simulink model "pd_lq_dob"  (Simulink 4.00)
settings: Solver=ode45  StartTime=0.0  StopTime=100.0  RelTol=1e-3
values from neighbouring files (symbols this model uses):
  B = 2.3006    [para_pdwithfriction.m]    (also in paradob.m)
  F_step = 0.1    [paradob.m]
  J = 2.7721    [para_pdwithfriction.m]    (also in paradob.m)
  Kp = 1    [para_pdwithfriction.m]    (also in paradob.m = 1.5)
  Kv = 0.02    [para_pdwithfriction.m]    (also in paradob.m)
  lqden = [ 1, -1.99971715402018,0.99972174296204,0,0,0]    [para_pdwithfriction.m]    (also in paradob.m = [1,-1.99630389598519,0.99631099777277,0,0,0])
  lqnum = 1000000*[1.50819599815358,-4.52194815122789,3.01001451018836,3.01970189465354,-4.52263469082776,1.50667043906476]    [para_pdwithfriction.m]    (also in paradob.m = 1000000*[0.99631443754708,-2.98490658969623,1.98438945750937)
  ts = 0.001    [para_pdwithfriction.m]    (also in paradob.m)
undefined symbols (not defined in the file or in its folder): g2den, g2num, qzden, qznum
libraries: simulink3 x1
settings Model: LastModifiedBy=liuyuan1  MaxDataPoints=100000  ExtModeTrigMode=oneshot  ExtModeArmWhenConnect=off

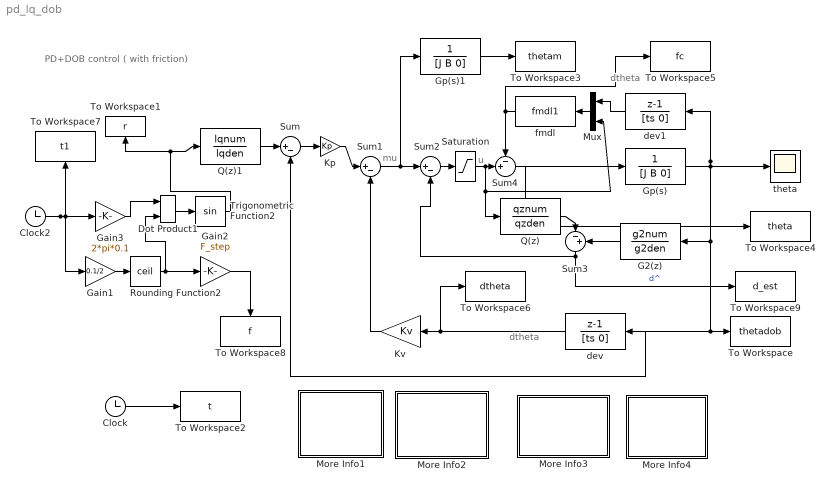
== system pd_lq_dob ==
  note: dtheta
  note: u
  note: PD+DOB control ( with friction)
  note: dtheta
  note: mu
  " Kv" : Gain  Orientation=left  Gain=Kv  Multiplication=Element-wise(K.*u)  SaturateOnIntegerOverflow=on
  Clock : Clock
      settings: DisplayTime=off  Decimation=10
  Clock2 : Clock
      settings: Decimation=10
  Dot Product1 : simulink3/Math/Dot Product
  G2(z) : DiscreteTransferFcn  Orientation=left  Numerator=g2num  Denominator=g2den  SampleTime=0.001  Realization=auto
      settings: RTWStateStorageClass=Auto
  Gain1 : Gain  Gain=0.1/2  Multiplication=Element-wise(K.*u)  SaturateOnIntegerOverflow=on
  Gain2 : Gain  Gain=F_step  Multiplication=Element-wise(K.*u)  SaturateOnIntegerOverflow=on
  Gain3 : Gain  Gain=2*pi*0.1  Multiplication=Element-wise(K.*u)  SaturateOnIntegerOverflow=on
  Gp(s) : TransferFcn  Numerator=[0 0 1]  Denominator=[J B 0]  AbsoluteTolerance=auto  Realization=auto
  Gp(s)1 : TransferFcn  Numerator=[0 0 1]  Denominator=[J B 0]  AbsoluteTolerance=auto  Realization=auto
  "Kp " : Gain  Gain=Kp  Multiplication=Element-wise(K.*u)  SaturateOnIntegerOverflow=on
  More Info1 : Subsystem
      settings: OpenFcn=eval(['paradob']);  RTWFcnNameOpts=Auto  RTWFileNameOpts=Auto
      mask Display: disp('Double click\nhere for\nload parameters')
  More Info2 : Subsystem
      settings: OpenFcn=eval(['postdobwithfriction']);  RTWFcnNameOpts=Auto  RTWFileNameOpts=Auto
      mask Display: disp('Double click\nhere for plot')
  More Info3 : Subsystem
      settings: OpenFcn=eval(['test_freq']);  RTWFcnNameOpts=Auto  RTWFileNameOpts=Auto
      mask Display: disp('Double click\nhere for \ncompute frequency')
  More Info4 : Subsystem
      settings: OpenFcn=eval(['bode_plot']);  RTWFcnNameOpts=Auto  RTWFileNameOpts=Auto
      mask Display: disp('Double click\nhere for \ndraw bode')
  Mux : Mux  Orientation=left  Inputs=2
  Q(z) : DiscreteTransferFcn  Numerator=qznum  Denominator=qzden  SampleTime=0.001  Realization=auto
      settings: RTWStateStorageClass=Auto
  Q(z)1 : DiscreteTransferFcn  Numerator=lqnum  Denominator=lqden  SampleTime=0.001  Realization=auto
      settings: RTWStateStorageClass=Auto
  Rounding Function2 : Rounding  Operator=ceil
  Saturation : Saturate  UpperLimit=10  LowerLimit=-10  LinearizeAsGain=on
  Sum : Sum  Inputs=|+-  SaturateOnIntegerOverflow=on
  Sum1 : Sum  Inputs=|+-  SaturateOnIntegerOverflow=on
  Sum2 : Sum  Inputs=|+-  SaturateOnIntegerOverflow=on
  Sum3 : Sum  Orientation=down  Inputs=|-+  SaturateOnIntegerOverflow=on
  Sum4 : Sum  Inputs=-+|  SaturateOnIntegerOverflow=on
  To Workspace : ToWorkspace  VariableName=thetadob  SampleTime=-1  SaveFormat=Array
      settings: MaxDataPoints=100000
  To Workspace1 : ToWorkspace  VariableName=r  SampleTime=-1  SaveFormat=Array
      settings: Orientation=up  MaxDataPoints=100000
  To Workspace2 : ToWorkspace  VariableName=t  SampleTime=-1  SaveFormat=Array
      settings: MaxDataPoints=100000
  To Workspace3 : ToWorkspace  VariableName=thetam  SampleTime=-1  SaveFormat=Array
      settings: MaxDataPoints=100000
  To Workspace4 : ToWorkspace  VariableName=theta  SampleTime=-1  SaveFormat=Array
      settings: MaxDataPoints=100000
  To Workspace5 : ToWorkspace  VariableName=fc  SampleTime=-1  SaveFormat=Array
      settings: MaxDataPoints=100000
  To Workspace6 : ToWorkspace  VariableName=dtheta  SampleTime=-1  SaveFormat=Array
      settings: MaxDataPoints=100000
  To Workspace7 : ToWorkspace  VariableName=t1  SampleTime=-1  SaveFormat=Array
      settings: Orientation=up
  To Workspace8 : ToWorkspace  VariableName=f  SampleTime=-1  SaveFormat=Array
      settings: Orientation=down  MaxDataPoints=100000
  To Workspace9 : ToWorkspace  VariableName=d_est  SampleTime=-1  SaveFormat=Array
      settings: MaxDataPoints=100000
  Trigonometric Function2 : Trigonometry  Operator=sin  OutputSignalType=auto
  dev : DiscreteTransferFcn  Orientation=left  Numerator=[1 -1]  Denominator=[ts 0]  SampleTime=0.001  Realization=auto
      settings: RTWStateStorageClass=Auto
  dev1 : DiscreteTransferFcn  Orientation=left  Numerator=[1 -1]  Denominator=[ts 0]  SampleTime=0.001  Realization=auto
      settings: RTWStateStorageClass=Auto
  fmdl : MATLABFcn  Orientation=left  MATLABFcn=fmdl1  OutputDimensions=-1  OutputSignalType=auto  Output1D=on
      settings: AttributesFormatString=fmdl2
  theta : Scope
      settings: TimeRange=auto  YMin=-1.5  YMax=1.5  SaveToWorkspace=off  SaveName=ScopeData  LimitDataPoints=on  MaxDataPoints=5000
  wires:
  Gp(s)/1 -> G2(z)/1, dev/1, Sum/2, To Workspace/1, dev1/1, theta/1, To Workspace4/1
  G2(z)/1 -> Sum3/2
  Q(z)/1 -> Sum3/1
  Sum/1 -> "Kp "/1
  "Kp "/1 -> Sum1/1
  " Kv"/1 -> Sum1/2
  Sum2/1 -> Saturation/1
  Sum4/1 -> Gp(s)/1
  Clock/1 -> To Workspace2/1
  Gp(s)1/1 -> To Workspace3/1
  Sum1/1 -> Sum2/1, Gp(s)1/1
  Sum3/1 -> To Workspace9/1, Sum2/2  "d^"
  fmdl/1 -> Sum4/1, To Workspace5/1
  Mux/1 -> fmdl/1
  dev1/1 -> Mux/1
  dev/1 -> " Kv"/1, To Workspace6/1
  Trigonometric Function2/1 -> To Workspace1/1, Q(z)1/1
  Clock2/1 -> Gain1/1, Gain3/1, To Workspace7/1
  Gain1/1 -> Rounding Function2/1
  Gain3/1 -> Dot Product1/1
  Rounding Function2/1 -> Dot Product1/2, Gain2/1
  Gain2/1 -> To Workspace8/1
  Saturation/1 -> Sum4/2, Q(z)/1, Mux/2
  Dot Product1/1 -> Trigonometric Function2/1
  Q(z)1/1 -> Sum/1

== system pd_lq_dob/More Info1 ==

== system pd_lq_dob/More Info2 ==

== system pd_lq_dob/More Info3 ==

== system pd_lq_dob/More Info4 ==
